simulink model "test2"  (R2021b)
settings: Solver=VariableStepAuto  StartTime=0.0  StopTime=10.0  RelTol=1e-3
libraries: canmsglib x2, SimulinkLibrary x1
settings Model: Creator=mujim  LastModifiedBy=mujim

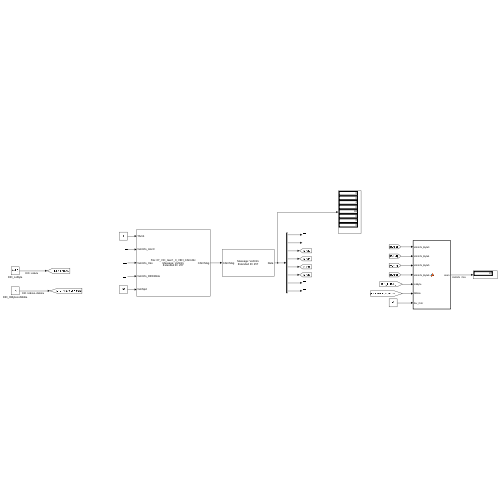
[thumbnail: Simulink's stored preview of the top-level diagram]
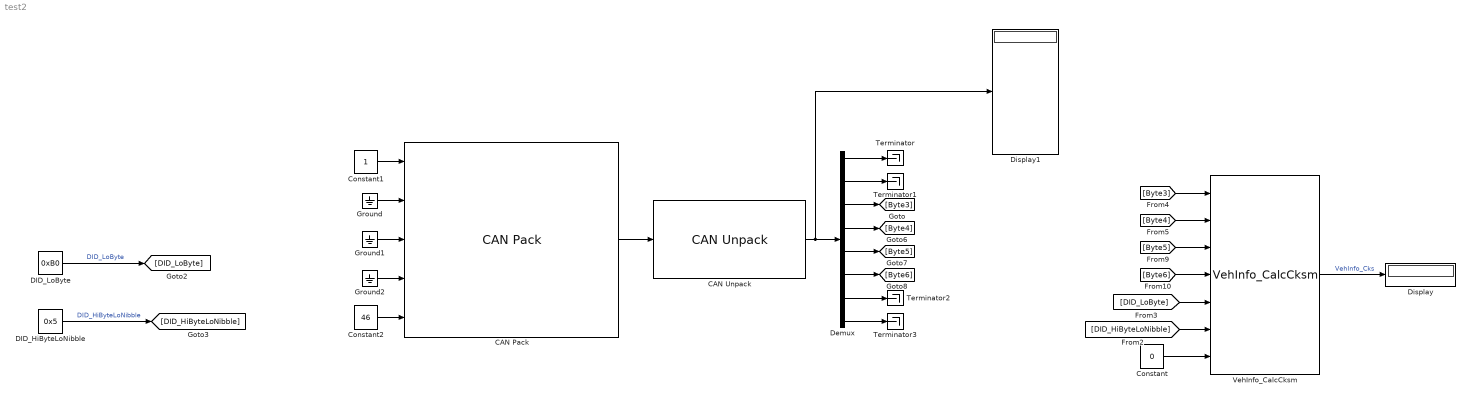
== system test2 ==
  CAN Pack : canmsglib/CAN Pack  CANdbFile=C:\Users\mujim\Kleanbus\Engineering - Documents\EV Bus\Components\Battery (Webasto)\batterys Notes\07_VIC_Gen1_0_VEH_CAN.dbc  MsgList=VehInfo  MsgName=VehInfo  MsgIDType=Extended (29-bit identifier)  MsgIdentifier=257  MsgLength=8  Remote=off  ApplyMinMax=off  BusOutput=off  SignalInfo={'TAmb','16','11','LE','signed','Standard','0','0.25','0','-256','255.75';'VehInfo_Alvctr','8','4','LE','unsigned','Standard','0','1','0','0','255';'VehInfo_Cks','0','8','LE','unsigned','Standard','0','1','0','0','255';'VehInfo_DIDNibble','12','4','LE','unsigned','Standard','0','1','0','0','255';'VehSpd','32','11','LE','signed','Standard','0','0.5','0','-512','511.5'}
      settings: SourceProductBaseCode=ME,XP,VN  DataFormat=CANdb specified signals
  CAN Unpack : canmsglib/CAN Unpack  MsgList=(none)  MsgName=VehInfo  MsgIDType=Extended (29-bit identifier)  MsgIdentifier=257  MsgLength=8  SignalInfo={}  IDPort=off  TimestampPort=off  ErrorPort=off  RemotePort=off  LengthPort=off  StatusPort=off  ApplyMinMax=off
      settings: SourceProductBaseCode=ME,XP,VN  DataFormat=raw data
  Constant : Constant  Value=0
  Constant1 : Constant
  Constant2 : Constant  Value=46
  DID_HiByteLoNibble : Constant  Value=0x5
  DID_LoByte : Constant  Value=0xB0
  Demux : Demux  Outputs=8
  Display : Display
  Display1 : Display
  Ground : Ground
  Ground1 : Ground
  Ground2 : Ground
  Terminator{,1..3} (4 alike) : Terminator
  VehInfo_CalcCksm : SimulinkLibrary/E2E_1C_VehInfo/VehInfo_CalcCksm  SystemSampleTime=-1  VariantActivationTime=update diagram  Latency=0  AutoFrameSizeCalculation=off
  wires:
  CAN Unpack/1 -> Display1/1, Demux/1
  DID_LoByte/1 -> [DID_LoByte]  "DID_LoByte"
  Constant1/1 -> CAN Pack/1
  CAN Pack/1 -> CAN Unpack/1
  Demux/8 -> Terminator3/1
  [DID_HiByteLoNibble] -> VehInfo_CalcCksm/6
  Ground/1 -> CAN Pack/2
  Constant2/1 -> CAN Pack/5
  Demux/7 -> Terminator2/1
  Demux/5 -> [Byte5]
  Ground2/1 -> CAN Pack/4
  [Byte3] -> VehInfo_CalcCksm/1
  Demux/4 -> [Byte4]
  DID_HiByteLoNibble/1 -> [DID_HiByteLoNibble]  "DID_HiByteLoNibble"
  Demux/3 -> [Byte3]
  Constant/1 -> VehInfo_CalcCksm/7
  Demux/2 -> Terminator1/1
  [Byte6] -> VehInfo_CalcCksm/4
  [DID_LoByte] -> VehInfo_CalcCksm/5
  [Byte4] -> VehInfo_CalcCksm/2
  Ground1/1 -> CAN Pack/3
  [Byte5] -> VehInfo_CalcCksm/3
  Demux/6 -> [Byte6]
  Demux/1 -> Terminator/1
  VehInfo_CalcCksm/1 -> Display/1  "VehInfo_Cks"
